simulink model "mass_spring_damper_RLS"  (R2019b)
settings: Solver=FixedStepAuto  StartTime=0.0  StopTime=50  FixedStep=0.01  RelTol=1e-3
settings Model: PacingRate=0.450000  Creator=Murray  LastModifiedBy=Murray

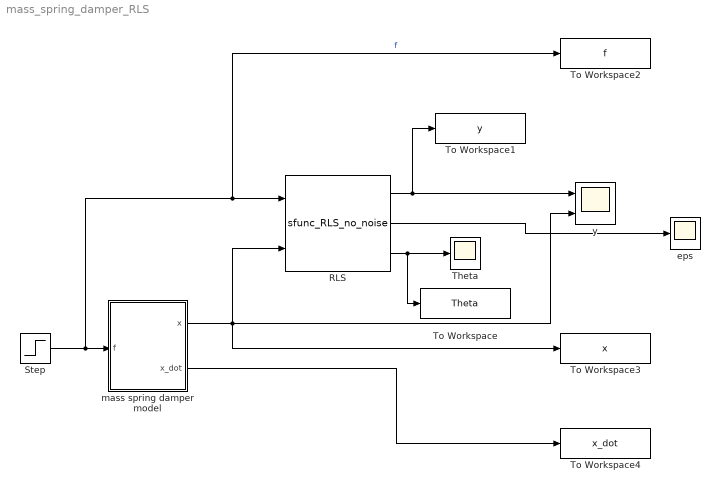
== system mass_spring_damper_RLS ==
  RLS : M-S-Function  FunctionName=sfunc_RLS_no_noise  Parameters=3, 0.999, 0.01
      mask Display:
      | port_label('input', 1, 'f')
      | port_label('input', 2, 'x')
      | port_label('output', 1, 'y')
      | port_label('output', 2, 'eps')
      | port_label('output', 3, 'Theta')
  Step : Step  SampleTime=0
  Theta : Scope
  To Workspace : ToWorkspace  VariableName=Theta  SaveFormat=Timeseries  SampleTime=-1
  To Workspace1 : ToWorkspace  VariableName=y  SaveFormat=Timeseries  SampleTime=-1
  To Workspace2 : ToWorkspace  VariableName=f  SaveFormat=Timeseries  SampleTime=-1
  To Workspace3 : ToWorkspace  VariableName=x  SaveFormat=Timeseries  SampleTime=-1
  To Workspace4 : ToWorkspace  VariableName=x_dot  SaveFormat=Timeseries  SampleTime=-1
  eps : Scope
  mass spring damper model : Subsystem
  y : Scope  NumInputPorts=2
  wires:
  Step/1 -> To Workspace2/1, RLS/1, mass spring damper model/1(f)  "f"
  mass spring damper model/1(x) -> y/2, RLS/2, To Workspace3/1
  RLS/1 -> To Workspace1/1, y/1
  RLS/2 -> eps/1
  RLS/3 -> To Workspace/1, Theta/1
  mass spring damper model/2(x_dot) -> To Workspace4/1

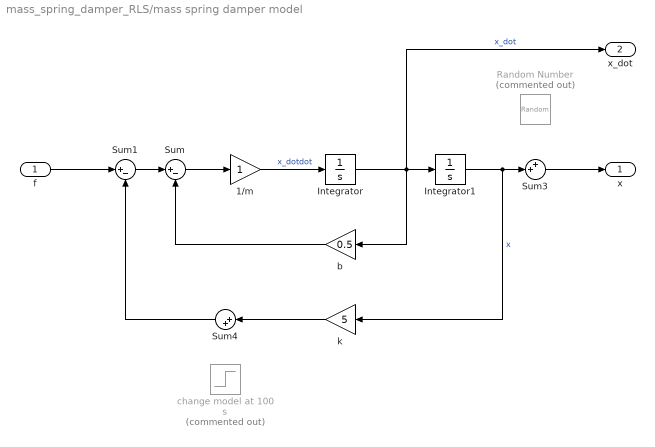
== system mass_spring_damper_RLS/mass spring damper model ==
  f : Inport
  1/m : Gain
  Integrator : Integrator
  Integrator1 : Integrator
  Random Number : RandomNumber  Commented=on  Variance=0.00001  Seed=1  SampleTime=0.01
  Sum : Sum  Inputs=|+-
  Sum1 : Sum  Inputs=|+-
  Sum3 : Sum  Inputs=++|
  Sum4 : Sum  Inputs=|++
  b : Gain  Gain=0.5
  change model at 100 s : Step  Commented=on  Time=100  SampleTime=0.01
  k : Gain  Gain=5
  x : Outport
  x_dot : Outport  Port=2
  wires:
  k/1 -> Sum4/1
  Sum4/1 -> Sum1/2
  Integrator1/1 -> Sum3/2, k/1  "x"
  f/1 -> Sum1/1
  Sum3/1 -> x/1
  Sum1/1 -> Sum/1
  Integrator/1 -> x_dot/1, b/1, Integrator1/1  "x_dot"
  Sum/1 -> 1/m/1
  1/m/1 -> Integrator/1  "x_dotdot"
  b/1 -> Sum/2
